simulink model "Differential"  (R2014a)
settings: Solver=ode45  StartTime=0.0  StopTime=10.0  RelTol=1e-3
undefined symbols (not defined in the file): l, phildot, phirdot, r, x0
libraries: simulink x1
settings Model: Creator=dariush  LastModifiedBy=dariush

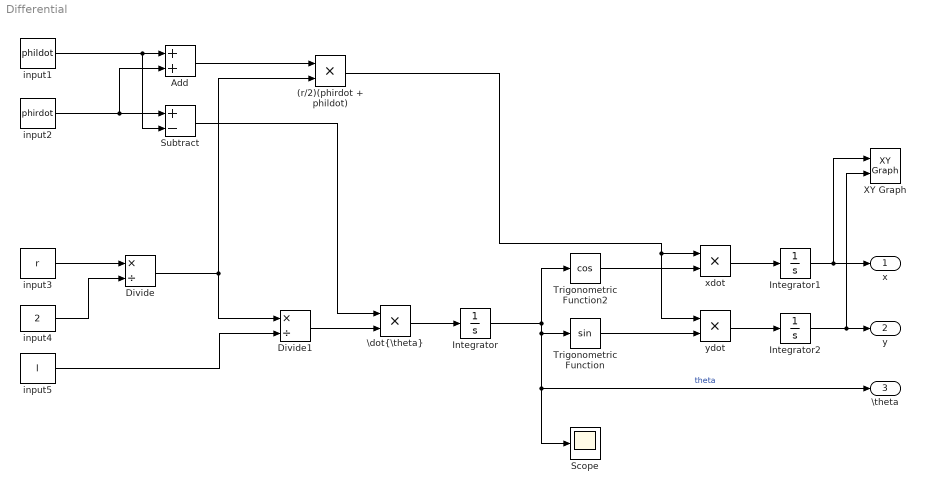
== system Differential ==
  (r/2)(phirdot + phildot) : Product
  Add : Sum
  Divide : Product  Inputs=*/
  Divide1 : Product  Inputs=*/
  Integrator : Integrator  InitialCondition=x0(3)
  Integrator1 : Integrator  InitialCondition=x0(1)
  Integrator2 : Integrator  InitialCondition=x0(2)
  Scope : Scope
      settings: TimeRange=10  YMin=0  YMax=25
  Subtract : Sum  Inputs=+-
  Trigonometric Function : Trigonometry
  Trigonometric Function2 : Trigonometry  Operator=cos
  XY Graph : simulink/Sinks/XY Graph  xmin=-1  xmax=1  ymin=-1  ymax=1  st=-1
  "\\dot{\\theta}" : Product
  input1 : Constant  Value=phildot
  input2 : Constant  Value=phirdot
  input3 : Constant  Value=r
  input4 : Constant  Value=2
  input5 : Constant  Value=l
  xdot : Product
  ydot : Product
  x : Outport
  y : Outport  Port=2
  \theta : Outport  Port=3
  wires:
  input1/1 -> Subtract/2, Add/1
  input2/1 -> Subtract/1, Add/2
  input3/1 -> Divide/1
  input4/1 -> Divide/2
  Divide/1 -> Divide1/1, (r/2)(phirdot + phildot)/2
  Add/1 -> (r/2)(phirdot + phildot)/1
  input5/1 -> Divide1/2
  Divide1/1 -> "\\dot{\\theta}"/2
  Subtract/1 -> "\\dot{\\theta}"/1
  "\\dot{\\theta}"/1 -> Integrator/1
  Integrator/1 -> Trigonometric Function2/1, \theta/1, Scope/1, Trigonometric Function/1  "theta"
  (r/2)(phirdot + phildot)/1 -> ydot/1, xdot/1
  Trigonometric Function2/1 -> xdot/2
  Trigonometric Function/1 -> ydot/2
  xdot/1 -> Integrator1/1
  Integrator1/1 -> XY Graph/1, x/1
  ydot/1 -> Integrator2/1
  Integrator2/1 -> XY Graph/2, y/1
